simulink model "LQR"  (R2016a)
settings: Solver=VariableStepAuto  SolverMode=SingleTasking  StartTime=0.0  StopTime=7.0  RelTol=1e-3
values from neighbouring files (symbols this model uses):
  A = [0 0 0 0 1 0 0 0; 0 0 0 0 0 1 0 0; 0 0 0 0 0 0 1 0; 0 0 0 0 0 0 0 1; temp(:,1:8)]    [inverted_pendulum_on_self_balancing_robot.m]
  B = [0 0; 0 0; 0 0; 0 0; temp(:,9:10)]    [inverted_pendulum_on_self_balancing_robot.m]
  K = dlqr(G,H,Q,R)    [inverted_pendulum_on_self_balancing_robot.m]
  x0 = [0; 0; -0.1745; 0.1745; 0; 0; 0; 0]    [inverted_pendulum_on_self_balancing_robot.m]
settings Model: Creator=Pascal  LastModifiedBy=WHEELTEC
settings DebuggingCC: SFUnexpectedBacktrackingDiag=error  SFNoUnconditionalDefaultTransitionDiag=error
settings SFSimCC: SimUseLocalCustomCode=on
settings RTWCC: RTWUseLocalCustomCode=on
settings GRTTargetCC: TargetLangStandard=C99 (ISO)
settings ConfigComp: CovMetricSettings=dwe  CovSaveCumulativeToWorkspaceVar=off  CovSaveSingleToWorkspaceVar=off  CovExternalEMLEnable=on

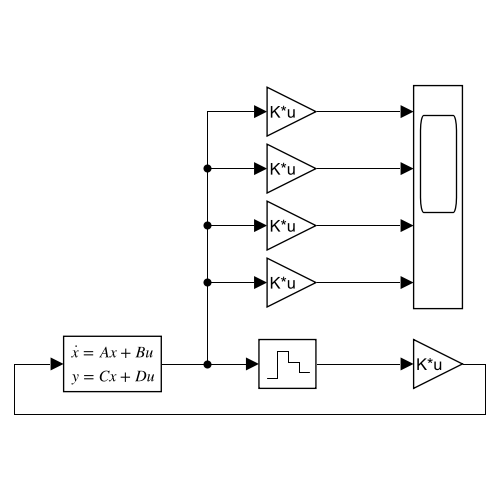
[thumbnail: Simulink's stored preview of the top-level diagram]
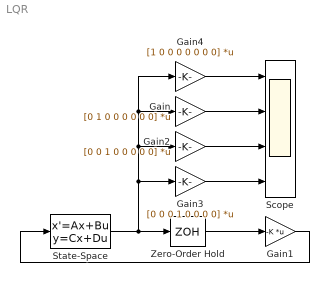
== system LQR ==
  Gain : Gain  Gain=[0 1 0 0 0 0 0 0]  Multiplication=Matrix(K*u)
  Gain1 : Gain  Gain=-K  Multiplication=Matrix(K*u)
  Gain2 : Gain  Gain=[0 0 1 0 0 0 0 0]  Multiplication=Matrix(K*u)
  Gain3 : Gain  Gain=[0 0 0 1 0 0 0 0]  Multiplication=Matrix(K*u)
  Gain4 : Gain  Gain=[1 0 0 0 0 0 0 0]  Multiplication=Matrix(K*u)
  Scope : Scope  NumInputPorts=4
  State-Space : StateSpace  A=A  B=B  C=eye(8)  D=zeros(8,2)  X0=x0
  Zero-Order Hold : ZeroOrderHold  SampleTime=0.01
  wires:
  State-Space/1 -> Gain4/1, Gain/1, Gain2/1, Gain3/1, Zero-Order Hold/1
  Zero-Order Hold/1 -> Gain1/1
  Gain1/1 -> State-Space/1
  Gain/1 -> Scope/2
  Gain2/1 -> Scope/3
  Gain3/1 -> Scope/4
  Gain4/1 -> Scope/1
